simulink model "bol1_ejer5_grafica2"  (R2021a)
settings: Solver=VariableStepAuto  StartTime=0.0  StopTime=10.0  RelTol=1e-3
settings Model: Creator=andrea  LastModifiedBy=andrea

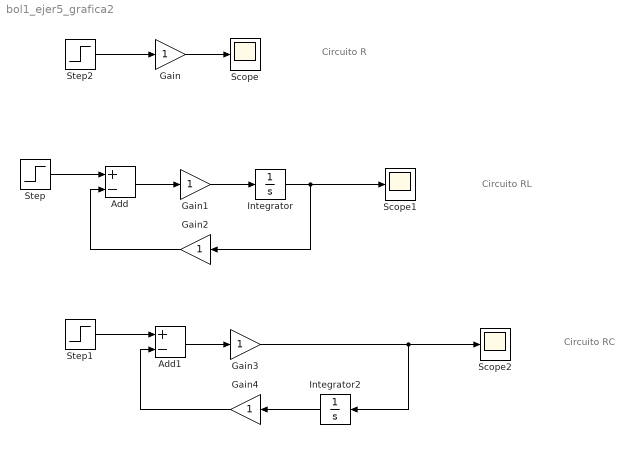
== system bol1_ejer5_grafica2 ==
  note: Circuito RL
  note: Circuito RC
  note: Circuito R
  Add : Sum  Inputs=+-
  Add1 : Sum  Inputs=+-
  Gain{,1..4} (5 alike) : Gain
  Integrator : Integrator
  Integrator2 : Integrator
  Scope : Scope
  Scope1 : Scope
  Scope2 : Scope
  Step : Step  SampleTime=0
  Step1 : Step  SampleTime=0
  Step2 : Step  SampleTime=0
  wires:
  Step2/1 -> Gain/1
  Gain1/1 -> Integrator/1
  Integrator/1 -> Gain2/1, Scope1/1
  Step/1 -> Add/1
  Add/1 -> Gain1/1
  Gain2/1 -> Add/2
  Add1/1 -> Gain3/1
  Gain4/1 -> Add1/2
  Step1/1 -> Add1/1
  Integrator2/1 -> Gain4/1
  Gain3/1 -> Integrator2/1, Scope2/1
  Gain/1 -> Scope/1
